simulink model "circuito"  (Simulink 7.7)
settings: Solver=ode3  StartTime=-0.05  StopTime=0.1  RelTol=1e-3
libraries: dspsigops x3
settings Model: Creator=ctu  LastModifiedBy=ctu

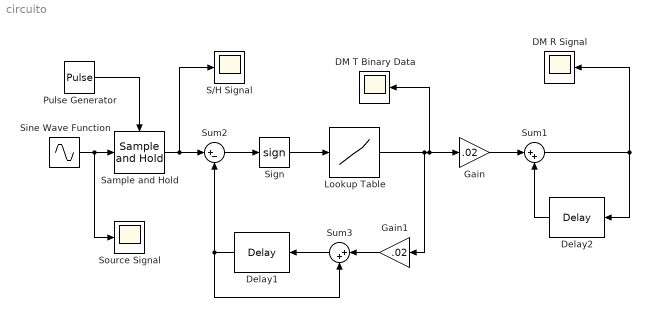
== system circuito ==
  DM R Signal : Scope
      settings: YMin=-1  YMax=1
  DM T Binary Data : Scope
      settings: YMin=-2  YMax=2  SaveName=ScopeData3
  Delay1 : dspsigops/Delay  InputProcessing=Inherited (this choice will be removed - see release notes)  dly_unit=Samples  delay=5  ic_detail=off  dif_ic_for_ch=off  dif_ic_for_dly=off  ic=0  reset_popup=None
  Delay2 : dspsigops/Delay  InputProcessing=Inherited (this choice will be removed - see release notes)  dly_unit=Samples  delay=5  ic_detail=off  dif_ic_for_ch=off  dif_ic_for_dly=off  ic=0  reset_popup=None
  Gain : Gain  Gain=.02
  Gain1 : Gain  Gain=.02
  Lookup Table : Lookup  InputValues=[-1,0,1]  Table=[-1,-1,1]  LookUpMeth=Use Input Nearest
  Pulse Generator : DiscretePulseGenerator  PulseType=Time based  Period=5e-4  PulseWidth=20
  S/H Signal : Scope
      settings: YMin=-1.5  YMax=1.5  SaveName=ScopeData2
  Sample and Hold : dspsigops/Sample and Hold  SystemSampleTime=-1  trig=Rising edge  initCond=0  latchinput=off
  Sign : Signum
  Sine Wave Function : Sin  Frequency=4*pi  SampleTime=1e-4
  Source Signal : Scope
      settings: YMin=-1.5  YMax=1.5
  Sum1 : Sum  Inputs=|++
  Sum2 : Sum  Inputs=|+-
  Sum3 : Sum  Inputs=|++
  wires:
  Sample and Hold/1 -> Sum2/1, S/H Signal/1
  Sum2/1 -> Sign/1
  Sign/1 -> Lookup Table/1
  Lookup Table/1 -> Gain1/1, Gain/1, DM T Binary Data/1
  Gain/1 -> Sum1/1
  Sum1/1 -> DM R Signal/1, Delay2/1
  Gain1/1 -> Sum3/1
  Sum3/1 -> Delay1/1
  Pulse Generator/1 -> Sample and Hold/Trigger
  Delay1/1 -> Sum2/2, Sum3/2
  Delay2/1 -> Sum1/2
  Sine Wave Function/1 -> Sample and Hold/1, Source Signal/1
